simulink model "uz_pmsm_model_old_commit"  (R2023b)
settings: Solver=FixedStepAuto  StartTime=0.0  StopTime=0.05  RelTol=1e-3
PreLoadFcn:
  | uz_pmsm_model_init_parameter
PostLoadFcn:
  | % Import the data from Excel for a lookup table
  | FluxMapData = readtable('C:\Users\Philipp\ultrazohm\ultrazohm_sw\ip_cores\uz_pmsm_model\FluxMapData_2023-05-26_13-07-57.csv');
  | % Row indices for lookup table
  | d_current_in_d_axis = FluxMapData(8:27,1:end);
  | % Column indices for lookup table
  | q_current_in_d_axis = FluxMapData(29:48,1:end);
  | % Output values for lookup table
  | d_Flux_d_axis = FluxMapData(50:69,1:end);
values from neighbouring files (symbols this model uses):
  ad1 = ad_1(1)    [LUT_approx_methode2a.m]    (also in LUT_approx_methode2a_clean.m = ad_self(1); LUT_approx_methode_2a_FEM.m; fitting_parameter.mat = 0.03048394862; fitting_parameter_48V_SynRM.mat = 0.0218446789236)
  ad2 = ad_1(2)    [LUT_approx_methode2a.m]    (also in LUT_approx_methode2a_clean.m = ad_self(2); LUT_approx_methode_2a_FEM.m; fitting_parameter.mat = 0.0402440194669; fitting_parameter_48V_SynRM.mat = 0.015691946268)
  ad3 = ad_1(3)    [LUT_approx_methode2a.m]    (also in LUT_approx_methode2a_clean.m = ad_self(3); LUT_approx_methode_2a_FEM.m; fitting_parameter.mat = -16.4812001193; fitting_parameter_48V_SynRM.mat = 2.77465564774)
  ad4 = ad_3_6(1)    [LUT_approx_methode2a.m]    (also in LUT_approx_methode2a_clean.m = ad_4_6(1); LUT_approx_methode_2a_FEM.m; fitting_parameter.mat = 1.2964378241; fitting_parameter_48V_SynRM.mat = 0.0214529395212)
  ad5 = ad_3_6(2)    [LUT_approx_methode2a.m]    (also in LUT_approx_methode2a_clean.m = ad_4_6(2); LUT_approx_methode_2a_FEM.m; fitting_parameter.mat = 0.000618316734858; fitting_parameter_48V_SynRM.mat = 0.0128514742508)
  ad6 = ad_3_6(3)    [LUT_approx_methode2a.m]    (also in LUT_approx_methode2a_clean.m = ad_4_6(3); LUT_approx_methode_2a_FEM.m; fitting_parameter.mat = -12.2755860444; fitting_parameter_48V_SynRM.mat = 2.54408267654)
  aq1 = aq_1(1)    [LUT_approx_methode2a.m]    (also in LUT_approx_methode2a_clean.m = aq_self(1); LUT_approx_methode_2a_FEM.m; fitting_parameter.mat = 0.0048166705291; fitting_parameter_48V_SynRM.mat = 0.00205546577039)
  aq2 = aq_1(2)    [LUT_approx_methode2a.m]    (also in LUT_approx_methode2a_clean.m = aq_self(2); LUT_approx_methode_2a_FEM.m; fitting_parameter.mat = 0.171595255564; fitting_parameter_48V_SynRM.mat = 0.0602932843871)
  aq3 = aq_1(3)    [LUT_approx_methode2a.m]    (also in LUT_approx_methode2a_clean.m = aq_self(3); LUT_approx_methode_2a_FEM.m; fitting_parameter.mat = 0.000926293864031; fitting_parameter_48V_SynRM.mat = 4.42738872822e-05)
  aq4 = aq_3_6(1)    [LUT_approx_methode2a.m]    (also in LUT_approx_methode2a_clean.m = aq_4_6(1); LUT_approx_methode_2a_FEM.m; fitting_parameter.mat = 0.00500187099075; fitting_parameter_48V_SynRM.mat = 0.000698420875152)
  aq5 = aq_3_6(2)    [LUT_approx_methode2a.m]    (also in LUT_approx_methode2a_clean.m = aq_4_6(2); LUT_approx_methode_2a_FEM.m; fitting_parameter.mat = 0.17052123489; fitting_parameter_48V_SynRM.mat = 0.0493122483219)
  aq6 = aq_3_6(3)    [LUT_approx_methode2a.m]    (also in LUT_approx_methode2a_clean.m = aq_4_6(3); LUT_approx_methode_2a_FEM.m; fitting_parameter.mat = 0.00091860845; fitting_parameter_48V_SynRM.mat = 4.14644316065e-05)
  d_current_d_Flux = FluxMapData{1,1:20}    [uz_pmsm_model_init_parameter.m]
  d_current_q_Flux = FluxMapData{66,1:20}    [uz_pmsm_model_init_parameter.m]
  entkopplung_dynamic = false    [compare_simulation_to_measurement.m]    (also in uz_pmsm_model_init_parameter.m; uz_pmsm_model_init_parameter_clean.m)
  entkopplung_linear = true    [compare_simulation_to_measurement.m]    (also in uz_pmsm_model_init_parameter.m = false; uz_pmsm_model_init_parameter_clean.m = false)
  entkopplung_static = false    [compare_simulation_to_measurement.m]    (also in uz_pmsm_model_init_parameter.m = true; uz_pmsm_model_init_parameter_clean.m)
  Fid1_Giq1 = ((1/2).*(aq3-aq6).*((q_current_set).^2))+((aq1./aq2).*log(cosh(aq2.*q_current_set)))-((aq4/aq5).*log(cosh(aq5.*q_current_set)))    [LUT_approx_methode2a.m]    (also in LUT_approx_methode2a_clean.m; LUT_approx_methode_2a_FEM.m = (1/2).*(aq3-aq6).*((q_current_set).^2)+((aq1./aq2).*log(cosh; fitting_parameter.mat = -0.00135679401385; fitting_parameter_48V_SynRM.mat = 0.221350145237)
  Fid2_Giq2 = ((ad1./ad2).*(log(cosh(ad2.*(d_current_set-ad3))))) - ((ad4./ad5).*(log(cosh(ad5.*(d_current_set-ad6)))))    [LUT_approx_methode2a.m]    (also in LUT_approx_methode2a_clean.m; LUT_approx_methode_2a_FEM.m = ((ad1./ad2).*(log(cosh(ad2.*(d_current_set-ad3))))) - (((ad1; fitting_parameter.mat = 0.0788137932988; fitting_parameter_48V_SynRM.mat = 0.221214979406)
  Flux_d = FluxMapData{43:62,1:20}'*(1e-3)    [uz_pmsm_model_init_parameter.m]
  Flux_q = FluxMapData{108:127,1:20}'*(1e-3)    [uz_pmsm_model_init_parameter.m]
  friction_coefficient = 0.001    [uz_pmsm_model_init_parameter.m]    (also in uz_pmsm_model_init_parameter_clean.m)
  inertia = 0.000084    (= 8.4e-05)    [uz_pmsm_model_init_parameter.m]    (also in uz_pmsm_model_init_parameter_clean.m)
  L_d = 0.3    [uz_pmsm_model_init_parameter.m]    (also in uz_pmsm_model_init_parameter_clean.m = 0.00045)
  L_q = 0.3    [uz_pmsm_model_init_parameter.m]    (also in uz_pmsm_model_init_parameter_clean.m = 0.002)
  load_torque = 0    [uz_pmsm_model_init_parameter.m]
  parameter_nachfuerung = false    [compare_simulation_to_measurement.m]    (also in uz_pmsm_model_init_parameter.m; uz_pmsm_model_init_parameter_clean.m)
  polepair = 4    [uz_pmsm_model_init_parameter.m]    (also in uz_pmsm_model_init_parameter_clean.m)
  praediktion_entkopplung_nonlinear = false    [compare_simulation_to_measurement.m]    (also in uz_pmsm_model_init_parameter.m; uz_pmsm_model_init_parameter_clean.m = true)
  psi_pm = 0.0075    [uz_pmsm_model_init_parameter.m]    (also in uz_pmsm_model_init_parameter_clean.m = 0.0194)
  q_current_d_Flux = FluxMapData{22:41,1}    [uz_pmsm_model_init_parameter.m]
  q_current_q_Flux = FluxMapData{87:106,1}    [uz_pmsm_model_init_parameter.m]
  R_1 = 0.08    [uz_pmsm_model_init_parameter.m]    (also in uz_pmsm_model_init_parameter_clean.m = 0.3)
  rpm = 1250    [uz_pmsm_model_init_parameter.m]
  setpoint_step = 4.0    (= 4)    [compare_simulation_to_measurement.m]    (also in export_csv.m = 10; iae_von_cil_measurements.m = 8; uz_pmsm_model_init_parameter.m = 8; uz_pmsm_model_init_parameter_clean.m = 10)
  simulate_mechanical = true    [compare_simulation_to_measurement.m]    (also in export_csv.m = false; uz_pmsm_model_init_parameter.m = false; uz_pmsm_model_init_parameter_clean.m = false)
  simulate_nonlinear_modell = false    [compare_simulation_to_measurement.m]    (also in uz_pmsm_model_init_parameter.m = true; uz_pmsm_model_init_parameter_clean.m = true)
  simulate_open_loop = true    [compare_simulation_to_measurement.m]    (also in export_csv.m; uz_pmsm_model_init_parameter.m = false; uz_pmsm_model_init_parameter_clean.m = false)
  static_friction_torque = 0.01    [uz_pmsm_model_init_parameter.m]    (also in uz_pmsm_model_init_parameter_clean.m)
  tau_sum = 2*ts_regler    (= 0.0001)    [uz_pmsm_model_init_parameter.m]    (also in uz_pmsm_model_init_parameter_clean.m = 8e-05)
  ts = logs{k}.Values    [export_csv.m]    (also in uz_pmsm_model_init_parameter.m = 2e-06; uz_pmsm_model_init_parameter_clean.m = 2e-06)
  ts_regler = 1/20e3    (= 5e-05)    [uz_pmsm_model_init_parameter.m]    (also in uz_pmsm_model_init_parameter_clean.m = 4e-05)
undefined symbols (not defined in the file or in its folder): Ki_Bo_d, Ki_Bo_q, Kp_Bo_d, Kp_Bo_q, Ldq
libraries: slpidlib x6
(part 4 of 5)

== system uz_pmsm_model_old_commit/Curren t_Controller_With_FluxMaps_OLD/Psi_d_q2/psid_approx ==
  Id : Inport
  Iq : Inport  Port=2
  FittingParameters : Inport  Port=3
  Demux : Demux  Outputs=23
  Log : Math  Operator=log  SignedPower=on
  Log1 : Math  Operator=log  SignedPower=on
  Product{,1..2,4..5,8} (6 alike) : Product  OutDataTypeStr=Inherit: Same as first input
  Product10 : Product  Inputs=3
  Product{3,6..7,12} (4 alike) : Product
  Sum : Sum  Inputs=|+-  OutDataTypeStr=Inherit: Same as first input
  Sum1 : Sum  Inputs=|+-
  Sum2 : Sum  Inputs=|+-  OutDataTypeStr=Inherit: Same as first input
  Sum3 : Sum  Inputs=|++-  OutDataTypeStr=Inherit: Same as first input
  Sum7 : Sum  Inputs=|+-  OutDataTypeStr=Inherit: Same as first input
  Tanh : Trigonometry  Operator=tanh
  Tanh1 : Trigonometry  Operator=tanh
  Tanh2 : Trigonometry  Operator=cosh
  Tanh3 : Trigonometry  Operator=cosh
  Terminator : Terminator
  psid : Outport
  psiq_cross_s1_integrated : Outport  Port=2
  wires:
  FittingParameters/1 -> Demux/1
  Demux/1 -> Product1/2  "ad1"
  Demux/3 -> Sum/2  "ad3"
  Sum/1 -> Product/1
  Demux/2 -> Product/2  "ad2"
  Product1/1 -> Sum7/1, Sum2/1  "psidself"
  Demux/4 -> Product3/2  "ad4"
  Sum1/1 -> Product2/1
  Demux/5 -> Product2/2  "ad5"
  Demux/6 -> Sum1/2  "ad6"
  Id/1 -> Sum1/1, Sum/1
  Product3/1 -> Sum2/2  "psid_s1"
  Iq/1 -> Product8/2, Product8/1, Product5/1, Product4/1
  Sum2/1 -> Product10/1  "psid_cross_s1"
  Tanh2/1 -> Log/1
  Tanh3/1 -> Log1/1
  Product8/1 -> Product7/1
  Product7/1 -> Sum3/2
  Demux/20 -> Product6/2
  Product6/1 -> Sum3/1
  Demux/19 -> Product12/2
  Product12/1 -> Sum3/3
  Sum3/1 -> Product10/2, psiq_cross_s1_integrated/1  "psiq_cross_s1_integrated"
  Demux/11 -> Product5/2  "aq5"
  Demux/8 -> Product4/2  "aq2"
  Product10/1 -> Sum7/2  "psid_cross"
  Sum7/1 -> psid/1  "psi_d_approx"
  Demux/14 -> Terminator/1
  Demux/13 -> Product10/3  "Reciprodical_F1G1"
  Log/1 -> Product6/1
  Log1/1 -> Product12/1
  Tanh/1 -> Product1/1
  Tanh1/1 -> Product3/1
  Product/1 -> Tanh/1
  Product2/1 -> Tanh1/1
  Product4/1 -> Tanh2/1
  Product5/1 -> Tanh3/1
  Demux/23 -> Product7/2

== system uz_pmsm_model_old_commit/Curren t_Controller_With_FluxMaps_OLD/Psi_d_q2/psid_approx1 ==
  Id : Inport
  Iq : Inport  Port=2
  FittingParameters : Inport  Port=3
  Demux : Demux  Outputs=23
  Log : Math  Operator=log  SignedPower=on
  Log1 : Math  Operator=log  SignedPower=on
  Product{,1..2,4..5,8} (6 alike) : Product  OutDataTypeStr=Inherit: Same as first input
  Product10 : Product  Inputs=3
  Product{3,6..7,12} (4 alike) : Product
  Sum : Sum  Inputs=|+-  OutDataTypeStr=Inherit: Same as first input
  Sum1 : Sum  Inputs=|+-
  Sum2 : Sum  Inputs=|+-  OutDataTypeStr=Inherit: Same as first input
  Sum3 : Sum  Inputs=|++-  OutDataTypeStr=Inherit: Same as first input
  Sum7 : Sum  Inputs=|+-  OutDataTypeStr=Inherit: Same as first input
  Tanh : Trigonometry  Operator=tanh
  Tanh1 : Trigonometry  Operator=tanh
  Tanh2 : Trigonometry  Operator=cosh
  Tanh3 : Trigonometry  Operator=cosh
  Terminator : Terminator
  psid : Outport
  psiq_cross_s1_integrated : Outport  Port=2
  wires:
  FittingParameters/1 -> Demux/1
  Demux/1 -> Product1/2  "ad1"
  Demux/3 -> Sum/2  "ad3"
  Sum/1 -> Product/1
  Demux/2 -> Product/2  "ad2"
  Product1/1 -> Sum7/1, Sum2/1  "psidself"
  Demux/4 -> Product3/2  "ad4"
  Sum1/1 -> Product2/1
  Demux/5 -> Product2/2  "ad5"
  Demux/6 -> Sum1/2  "ad6"
  Id/1 -> Sum1/1, Sum/1
  Product3/1 -> Sum2/2  "psid_s1"
  Iq/1 -> Product8/2, Product8/1, Product5/1, Product4/1
  Sum2/1 -> Product10/1  "psid_cross_s1"
  Tanh2/1 -> Log/1
  Tanh3/1 -> Log1/1
  Product8/1 -> Product7/1
  Product7/1 -> Sum3/2
  Demux/20 -> Product6/2
  Product6/1 -> Sum3/1
  Demux/19 -> Product12/2
  Product12/1 -> Sum3/3
  Sum3/1 -> Product10/2, psiq_cross_s1_integrated/1  "psiq_cross_s1_integrated"
  Demux/11 -> Product5/2  "aq5"
  Demux/8 -> Product4/2  "aq2"
  Product10/1 -> Sum7/2  "psid_cross"
  Sum7/1 -> psid/1  "psi_d_approx"
  Demux/14 -> Terminator/1
  Demux/13 -> Product10/3  "Reciprodical_F1G1"
  Log/1 -> Product6/1
  Log1/1 -> Product12/1
  Tanh/1 -> Product1/1
  Tanh1/1 -> Product3/1
  Product/1 -> Tanh/1
  Product2/1 -> Tanh1/1
  Product4/1 -> Tanh2/1
  Product5/1 -> Tanh3/1
  Demux/23 -> Product7/2

== system uz_pmsm_model_old_commit/Curren t_Controller_With_FluxMaps_OLD/Psi_d_q2/psiq_approx ==
  Id : Inport
  Iq : Inport  Port=2
  FittingParameters : Inport  Port=3
  Demux : Demux  Outputs=23
  Log1 : Math  Operator=log  SignedPower=on
  Log2 : Math  Operator=log  SignedPower=on
  Product{,2,7,10} (4 alike) : Product  OutDataTypeStr=Inherit: Same as first input
  Product{1,3..6,9} (6 alike) : Product
  Product20 : Product  Inputs=3
  Sum1 : Sum  Inputs=|++
  Sum10 : Sum  Inputs=|+-
  Sum2 : Sum  Inputs=|+-
  Sum3 : Sum  Inputs=-+|
  Sum4 : Sum  Inputs=++|
  Sum5 : Sum  Inputs=|+-
  Sum6 : Sum  Inputs=-+|
  Tanh : Trigonometry  Operator=tanh
  Tanh1 : Trigonometry  Operator=tanh
  Tanh2 : Trigonometry  Operator=cosh
  Tanh4 : Trigonometry  Operator=cosh
  psiq : Outport
  psid_cross_s1_integrated : Outport  Port=2
  wires:
  FittingParameters/1 -> Demux/1
  Sum2/1 -> Product20/1  "psiq_cross_s1"
  Demux/10 -> Product3/2  "aq4"
  Demux/12 -> Product6/2  "aq6"
  Demux/8 -> Product/2  "aq2"
  Demux/11 -> Product2/2  "aq5"
  Demux/7 -> Product1/2  "aq1"
  Iq/1 -> Product2/1, Product6/1, Product/1, Product5/1
  Demux/9 -> Product5/2  "aq3"
  Tanh4/1 -> Log2/1
  Demux/22 -> Product4/1
  Product1/1 -> Sum4/2
  Product5/1 -> Sum4/1
  Sum4/1 -> Sum10/1, Sum2/1  "psiq_self"
  Sum1/1 -> Sum2/2
  Product3/1 -> Sum1/1  "psiq_s1"
  Product6/1 -> Sum1/2
  Sum3/1 -> Product7/2  "psid_cross_s1"
  Product7/1 -> Tanh4/1  "psid_s1"
  Product4/1 -> Sum5/1
  Product9/1 -> Sum5/2
  Product10/1 -> Tanh2/1  "psid_s1"
  Tanh2/1 -> Log1/1
  Demux/21 -> Product9/1
  Sum6/1 -> Product10/2  "psid_cross_s1"
  Demux/3 -> Sum3/1  "ad3"
  Demux/2 -> Product7/1  "ad2"
  Demux/5 -> Product10/1  "ad5"
  Demux/6 -> Sum6/1  "ad6"
  Id/1 -> Sum6/2, Sum3/2
  Sum5/1 -> psid_cross_s1_integrated/1, Product20/2  "psid_cross_s1_integrated"
  Product20/1 -> Sum10/2  "psiq_cross"
  Sum10/1 -> psiq/1  "psiq_approx"
  Demux/14 -> Product20/3
  Log1/1 -> Product9/2
  Log2/1 -> Product4/2
  Tanh1/1 -> Product3/1
  Tanh/1 -> Product1/1
  Product2/1 -> Tanh1/1
  Product/1 -> Tanh/1

== system uz_pmsm_model_old_commit/Curren t_Controller_With_FluxMaps_OLD/Psi_d_q2/psiq_approx1 ==
  Id : Inport
  Iq : Inport  Port=2
  FittingParameters : Inport  Port=3
  Demux : Demux  Outputs=23
  Log1 : Math  Operator=log  SignedPower=on
  Log2 : Math  Operator=log  SignedPower=on
  Product{,2,7,10} (4 alike) : Product  OutDataTypeStr=Inherit: Same as first input
  Product{1,3..6,9} (6 alike) : Product
  Product20 : Product  Inputs=3
  Sum1 : Sum  Inputs=|++
  Sum10 : Sum  Inputs=|+-  OutDataTypeStr=Inherit: Same as first input
  Sum2 : Sum  Inputs=|+-
  Sum3 : Sum  Inputs=-+|
  Sum4 : Sum  Inputs=++|
  Sum5 : Sum  Inputs=|+-
  Sum6 : Sum  Inputs=-+|
  Tanh : Trigonometry  Operator=tanh
  Tanh1 : Trigonometry  Operator=tanh
  Tanh2 : Trigonometry  Operator=cosh
  Tanh4 : Trigonometry  Operator=cosh
  psiq : Outport
  psid_cross_s1_integrated : Outport  Port=2
  wires:
  FittingParameters/1 -> Demux/1
  Sum2/1 -> Product20/1  "psiq_cross_s1"
  Demux/10 -> Product3/2  "aq4"
  Demux/12 -> Product6/2  "aq6"
  Demux/8 -> Product/2  "aq2"
  Demux/11 -> Product2/2  "aq5"
  Demux/7 -> Product1/2  "aq1"
  Iq/1 -> Product2/1, Product6/1, Product/1, Product5/1
  Demux/9 -> Product5/2  "aq3"
  Tanh4/1 -> Log2/1
  Demux/22 -> Product4/1
  Product1/1 -> Sum4/2
  Product5/1 -> Sum4/1
  Sum4/1 -> Sum10/1, Sum2/1  "psiq_self"
  Sum1/1 -> Sum2/2
  Product3/1 -> Sum1/1  "psiq_s1"
  Product6/1 -> Sum1/2
  Sum3/1 -> Product7/2  "psid_cross_s1"
  Product7/1 -> Tanh4/1  "psid_s1"
  Product4/1 -> Sum5/1
  Product9/1 -> Sum5/2
  Product10/1 -> Tanh2/1  "psid_s1"
  Tanh2/1 -> Log1/1
  Demux/21 -> Product9/1
  Sum6/1 -> Product10/2  "psid_cross_s1"
  Demux/3 -> Sum3/1  "ad3"
  Demux/2 -> Product7/1  "ad2"
  Demux/5 -> Product10/1  "ad5"
  Demux/6 -> Sum6/1  "ad6"
  Id/1 -> Sum6/2, Sum3/2
  Sum5/1 -> psid_cross_s1_integrated/1, Product20/2  "psid_cross_s1_integrated"
  Product20/1 -> Sum10/2  "psiq_cross"
  Sum10/1 -> psiq/1  "psiq_approx"
  Demux/14 -> Product20/3
  Log1/1 -> Product9/2
  Log2/1 -> Product4/2
  Tanh1/1 -> Product3/1
  Tanh/1 -> Product1/1
  Product2/1 -> Tanh1/1
  Product/1 -> Tanh/1

== system uz_pmsm_model_old_commit/Current_Controller1/Entkopplungen/Lineare_Entkopplung ==
  i_d : Inport
  i_q : Inport  Port=2
  omega_m : Inport  Port=3
  Constant1 : Constant  Value=psi_pm  OutDataTypeStr=Inherit: Inherit via back propagation  SampleTime=-1
  Gain : Gain  Gain=L_q
  Gain1 : Gain  Gain=L_d
  Gain2 : Gain  Gain=polepair  OutDataTypeStr=Inherit: Same as input
  Product : Product  OutDataTypeStr=Inherit: Same as first input
  Product1 : Product  OutDataTypeStr=Inherit: Same as first input
  Sum6 : Sum  Inputs=|++
  u_d : Outport
  u_q : Outport  Port=2
  wires:
  omega_m/1 -> Gain2/1
  Sum6/1 -> Product1/1
  Product/1 -> u_d/1
  i_d/1 -> Gain1/1
  i_q/1 -> Gain/1
  Product1/1 -> u_q/1
  Gain1/1 -> Sum6/1
  Gain2/1 -> Product1/2, Product/2
  Gain/1 -> Product/1
  Constant1/1 -> Sum6/2  "u_q"

== system uz_pmsm_model_old_commit/Current_Controller1/Entkopplungen/decoupling_praediktion ==
  i_d : Inport
  u_d_1 : Inport  Port=2
  i_q : Inport  Port=3
  u_q_1 : Inport  Port=4
  omega_m : Inport  Port=5
  u_d_k : Inport  Port=6
  u_q_k : Inport  Port=7
  psi_q : Inport  Port=8
  psi_d : Inport  Port=9
  Gain : Gain  Gain=R_1
  Gain1 : Gain  Gain=R_1
  Gain2 : Gain  Gain=polepair
  Gain3 : Gain  Gain=ts_regler
  Gain4 : Gain  Gain=ts_regler
  Gain5 : Gain  Gain=ts_regler/2
  Gain6 : Gain  Gain=ts_regler/2
  Product{1..4} (4 alike) : Product
  Sum : Sum  Inputs=|+-
  Sum1 : Sum  Inputs=|+-
  Sum2 : Sum  Inputs=++|
  Sum3 : Sum  Inputs=|-+
  Sum4 : Sum  Inputs=++|
  Sum5 : Sum  Inputs=|++
  Sum6 : Sum  Inputs=++|
  Sum7 : Sum  Inputs=|++
  u_d_entk : Outport
  u_q_entk : Outport  Port=2
  wires:
  psi_q/1 -> Sum5/2, Product2/1
  psi_d/1 -> Product3/2, Sum4/1
  Gain2/1 -> Product1/2, Product4/1, Product3/1, Product2/2
  u_d_k/1 -> Sum/2
  Gain/1 -> Sum/1
  u_q_k/1 -> Sum1/1
  Gain1/1 -> Sum1/2
  Product3/1 -> Sum3/1
  Product2/1 -> Sum2/2
  Sum/1 -> Sum2/1
  Sum1/1 -> Sum3/2
  Sum3/1 -> Gain4/1
  Sum2/1 -> Gain3/1
  Gain3/1 -> Sum4/2
  Gain4/1 -> Sum5/1
  u_d_1/1 -> Gain5/1
  Sum4/1 -> Sum6/2
  u_q_1/1 -> Gain6/1
  Gain5/1 -> Sum6/1
  Sum5/1 -> Sum7/1
  Gain6/1 -> Sum7/2
  Sum6/1 -> Product1/1
  Sum7/1 -> Product4/2
  omega_m/1 -> Gain2/1
  i_d/1 -> Gain/1
  i_q/1 -> Gain1/1
  Product1/1 -> u_q_entk/1
  Product4/1 -> u_d_entk/1

== system uz_pmsm_model_old_commit/Current_Controller1/Entkopplungen/dynamic_nonlinear_entkopplung1 ==
  i_d : Inport
  i_q : Inport  Port=2
  psi_d : Inport  Port=3
  psi_q : Inport  Port=4
  Ldq_LUT : Inport  Port=5
  Lqd_LUT : Inport  Port=6
  omega_m : Inport  Port=7
  Gain2 : Gain  Gain=polepair
  Product : Product  OutDataTypeStr=Inherit: Same as first input
  Product1 : Product  OutDataTypeStr=Inherit: Same as first input
  Product2 : Product
  Product3 : Product
  Sum1 : Sum  Inputs=++|  OutDataTypeStr=Inherit: Same as first input
  Sum6 : Sum  Inputs=++|
  u_d : Outport
  u_q : Outport  Port=2
  wires:
  psi_q/1 -> Product/1  "psi_q_LUT"
  Gain2/1 -> Product1/2, Product/2
  psi_d/1 -> Product1/1  "psi_d_LUT"
  omega_m/1 -> Gain2/1
  i_d/1 -> Product2/1
  Ldq_LUT/1 -> Product2/2
  Sum6/1 -> u_q/1
  Product1/1 -> Sum6/2
  Product/1 -> Sum1/2
  Sum1/1 -> u_d/1
  i_q/1 -> Product3/1
  Lqd_LUT/1 -> Product3/2
  Product3/1 -> Sum6/1
  Product2/1 -> Sum1/1

== system uz_pmsm_model_old_commit/Current_Controller1/Entkopplungen/static_nonlinear_entkopplung ==
  psi_d : Inport
  psi_q : Inport  Port=2
  omega_m : Inport  Port=3
  Gain2 : Gain  Gain=polepair
  Product : Product  OutDataTypeStr=Inherit: Same as first input
  Product1 : Product  OutDataTypeStr=Inherit: Same as first input
  u_d : Outport
  u_q : Outport  Port=2
  wires:
  psi_q/1 -> Product/1  "psi_q_LUT"
  Gain2/1 -> Product1/2, Product/2
  Product1/1 -> u_q/1
  Product/1 -> u_d/1
  psi_d/1 -> Product1/1  "psi_d_LUT"
  omega_m/1 -> Gain2/1

== system uz_pmsm_model_old_commit/Current_Controller1/Psi_d_q1/Ldd_approx1 ==
  psiq_cross_s1_integrated : Inport
  Id : Inport  Port=2
  FittingParameters : Inport  Port=3
  Demux : Demux  Outputs=23
  Product{,1..3} (4 alike) : Product  OutDataTypeStr=single
  Product10 : Product  Inputs=3  OutDataTypeStr=single
  Product14 : Product
  Product15 : Product
  Reciprocal : Product  Inputs=/  RndMeth=Zero  SaturateOnIntegerOverflow=on
  Reciprocal1 : Product  Inputs=/  RndMeth=Zero  SaturateOnIntegerOverflow=on
  Sum : Sum  Inputs=|+-  OutDataTypeStr=single
  Sum1 : Sum  Inputs=|+-  OutDataTypeStr=single
  Sum2 : Sum  Inputs=|+-
  Sum7 : Sum  Inputs=|+-
  Tanh1 : Trigonometry  Operator=cosh
  Tanh4 : Trigonometry  Operator=cosh
  Ldd : Outport
  wires:
  FittingParameters/1 -> Demux/1
  Demux/3 -> Sum/2  "ad3"
  Sum/1 -> Product/1
  Demux/2 -> Product/2  "ad2"
  Product1/1 -> Sum7/1, Sum2/1  "psidself_abgeleitet"
  Sum1/1 -> Product2/1
  Demux/5 -> Product2/2  "ad5"
  Demux/6 -> Sum1/2  "ad6"
  Id/1 -> Sum1/1, Sum/1
  Product3/1 -> Sum2/2  "psid_s1"
  Sum2/1 -> Product10/1  "psid_cross_s1_abgeleitet"
  Product10/1 -> Sum7/2  "psid_cross"
  Sum7/1 -> Ldd/1  "psid_cross_s1"
  Demux/13 -> Product10/3  "F1G1"
  Tanh4/1 -> Product14/1, Product14/2
  Tanh1/1 -> Product15/2, Product15/1
  Reciprocal1/1 -> Product3/1
  Product15/1 -> Reciprocal1/1
  Product14/1 -> Reciprocal/1
  Product/1 -> Tanh4/1
  Product2/1 -> Tanh1/1
  psiq_cross_s1_integrated/1 -> Product10/2
  Reciprocal/1 -> Product1/1
  Demux/15 -> Product3/2  "ad4*ad5"
  Demux/16 -> Product1/2  "ad1*ad2"

== system uz_pmsm_model_old_commit/Current_Controller1/Psi_d_q1/Lqq_approx1 ==
  psid_cross_s1_integrated : Inport
  Iq : Inport  Port=2
  FittingParameters : Inport  Port=3
  Demux : Demux  Outputs=23
  Product : Product  OutDataTypeStr=Inherit: Same as first input
  Product1 : Product
  Product14 : Product  OutDataTypeStr=Inherit: Same as first input
  Product15 : Product
  Product2 : Product  OutDataTypeStr=Inherit: Same as first input
  Product20 : Product  Inputs=3
  Product3 : Product
  Reciprocal : Product  Inputs=/  RndMeth=Zero  SaturateOnIntegerOverflow=on
  Reciprocal1 : Product  Inputs=/  RndMeth=Zero  SaturateOnIntegerOverflow=on
  Sum1 : Sum  Inputs=|++
  Sum10 : Sum  Inputs=|+-
  Sum2 : Sum  Inputs=|+-
  Sum4 : Sum  Inputs=|++
  Tanh1 : Trigonometry  Operator=cosh
  Tanh3 : Trigonometry  Operator=cosh
  Lqq : Outport
  wires:
  FittingParameters/1 -> Demux/1
  Demux/12 -> Sum4/2  "aq6"
  Product20/1 -> Sum10/2  "psiq_cross"
  Sum10/1 -> Lqq/1  "Lqq"
  Demux/14 -> Product20/3
  Demux/9 -> Sum1/2  "aq3"
  Tanh3/1 -> Product14/1, Product14/2
  Tanh1/1 -> Product15/2, Product15/1
  Sum2/1 -> Product20/1
  Reciprocal/1 -> Product1/1
  Reciprocal1/1 -> Product3/1
  Demux/8 -> Product/2  "aq2"
  Iq/1 -> Product2/1, Product/1
  Demux/11 -> Product2/2  "aq5"
  Product1/1 -> Sum1/1  "psidself_abgeleitet"
  Sum1/1 -> Sum10/1, Sum2/1
  Sum4/1 -> Sum2/2
  Product3/1 -> Sum4/1  "psid_s1"
  Product15/1 -> Reciprocal1/1
  Product2/1 -> Tanh1/1
  Product/1 -> Tanh3/1
  Product14/1 -> Reciprocal/1
  psid_cross_s1_integrated/1 -> Product20/2
  Demux/18 -> Product1/2  "aq1*aq2"
  Demux/17 -> Product3/2  "aq4*aq5"

== system uz_pmsm_model_old_commit/Current_Controller1/Psi_d_q1/psid_approx ==
  Id : Inport
  Iq : Inport  Port=2
  FittingParameters : Inport  Port=3
  Demux : Demux  Outputs=23
  Log : Math  Operator=log  SignedPower=on
  Log1 : Math  Operator=log  SignedPower=on
  Product{,1..2,4..5,8} (6 alike) : Product  OutDataTypeStr=Inherit: Same as first input
  Product10 : Product  Inputs=3
  Product{3,6..7,12} (4 alike) : Product
  Sum : Sum  Inputs=|+-  OutDataTypeStr=Inherit: Same as first input
  Sum1 : Sum  Inputs=|+-
  Sum2 : Sum  Inputs=|+-  OutDataTypeStr=Inherit: Same as first input
  Sum3 : Sum  Inputs=|++-  OutDataTypeStr=Inherit: Same as first input
  Sum7 : Sum  Inputs=|+-  OutDataTypeStr=Inherit: Same as first input
  Tanh : Trigonometry  Operator=tanh
  Tanh1 : Trigonometry  Operator=tanh
  Tanh2 : Trigonometry  Operator=cosh
  Tanh3 : Trigonometry  Operator=cosh
  Terminator : Terminator
  psid : Outport
  psiq_cross_s1_integrated : Outport  Port=2
  wires:
  FittingParameters/1 -> Demux/1
  Demux/1 -> Product1/2  "ad1"
  Demux/3 -> Sum/2  "ad3"
  Sum/1 -> Product/1
  Demux/2 -> Product/2  "ad2"
  Product1/1 -> Sum7/1, Sum2/1  "psidself"
  Demux/4 -> Product3/2  "ad4"
  Sum1/1 -> Product2/1
  Demux/5 -> Product2/2  "ad5"
  Demux/6 -> Sum1/2  "ad6"
  Id/1 -> Sum1/1, Sum/1
  Product3/1 -> Sum2/2  "psid_s1"
  Iq/1 -> Product8/2, Product8/1, Product5/1, Product4/1
  Sum2/1 -> Product10/1  "psid_cross_s1"
  Tanh2/1 -> Log/1
  Tanh3/1 -> Log1/1
  Product8/1 -> Product7/1
  Product7/1 -> Sum3/2
  Demux/20 -> Product6/2
  Product6/1 -> Sum3/1
  Demux/19 -> Product12/2
  Product12/1 -> Sum3/3
  Sum3/1 -> Product10/2, psiq_cross_s1_integrated/1  "psiq_cross_s1_integrated"
  Demux/11 -> Product5/2  "aq5"
  Demux/8 -> Product4/2  "aq2"
  Product10/1 -> Sum7/2  "psid_cross"
  Sum7/1 -> psid/1  "psi_d_approx"
  Demux/14 -> Terminator/1
  Demux/13 -> Product10/3  "Reciprodical_F1G1"
  Log/1 -> Product6/1
  Log1/1 -> Product12/1
  Tanh/1 -> Product1/1
  Tanh1/1 -> Product3/1
  Product/1 -> Tanh/1
  Product2/1 -> Tanh1/1
  Product4/1 -> Tanh2/1
  Product5/1 -> Tanh3/1
  Demux/23 -> Product7/2

== system uz_pmsm_model_old_commit/Current_Controller1/Psi_d_q1/psiq_approx ==
  Id : Inport
  Iq : Inport  Port=2
  FittingParameters : Inport  Port=3
  Demux : Demux  Outputs=23
  Log1 : Math  Operator=log  SignedPower=on
  Log2 : Math  Operator=log  SignedPower=on
  Product{,2,7,10} (4 alike) : Product  OutDataTypeStr=Inherit: Same as first input
  Product{1,3..6,9} (6 alike) : Product
  Product20 : Product  Inputs=3
  Sum1 : Sum  Inputs=|++
  Sum10 : Sum  Inputs=|+-
  Sum2 : Sum  Inputs=|+-
  Sum3 : Sum  Inputs=-+|
  Sum4 : Sum  Inputs=++|
  Sum5 : Sum  Inputs=|+-
  Sum6 : Sum  Inputs=-+|
  Tanh : Trigonometry  Operator=tanh
  Tanh1 : Trigonometry  Operator=tanh
  Tanh2 : Trigonometry  Operator=cosh
  Tanh4 : Trigonometry  Operator=cosh
  psiq : Outport
  psid_cross_s1_integrated : Outport  Port=2
  wires:
  FittingParameters/1 -> Demux/1
  Sum2/1 -> Product20/1  "psiq_cross_s1"
  Demux/10 -> Product3/2  "aq4"
  Demux/12 -> Product6/2  "aq6"
  Demux/8 -> Product/2  "aq2"
  Demux/11 -> Product2/2  "aq5"
  Demux/7 -> Product1/2  "aq1"
  Iq/1 -> Product2/1, Product6/1, Product/1, Product5/1
  Demux/9 -> Product5/2  "aq3"
  Tanh4/1 -> Log2/1
  Demux/22 -> Product4/1
  Product1/1 -> Sum4/2
  Product5/1 -> Sum4/1
  Sum4/1 -> Sum10/1, Sum2/1  "psiq_self"
  Sum1/1 -> Sum2/2
  Product3/1 -> Sum1/1  "psiq_s1"
  Product6/1 -> Sum1/2
  Sum3/1 -> Product7/2  "psid_cross_s1"
  Product7/1 -> Tanh4/1  "psid_s1"
  Product4/1 -> Sum5/1
  Product9/1 -> Sum5/2
  Product10/1 -> Tanh2/1  "psid_s1"
  Tanh2/1 -> Log1/1
  Demux/21 -> Product9/1
  Sum6/1 -> Product10/2  "psid_cross_s1"
  Demux/3 -> Sum3/1  "ad3"
  Demux/2 -> Product7/1  "ad2"
  Demux/5 -> Product10/1  "ad5"
  Demux/6 -> Sum6/1  "ad6"
  Id/1 -> Sum6/2, Sum3/2
  Sum5/1 -> psid_cross_s1_integrated/1, Product20/2  "psid_cross_s1_integrated"
  Product20/1 -> Sum10/2  "psiq_cross"
  Sum10/1 -> psiq/1  "psiq_approx"
  Demux/14 -> Product20/3
  Log1/1 -> Product9/2
  Log2/1 -> Product4/2
  Tanh1/1 -> Product3/1
  Tanh/1 -> Product1/1
  Product2/1 -> Tanh1/1
  Product/1 -> Tanh/1

== system uz_pmsm_model_old_commit/Current_Controller_With_FluxMaps_OLD1/Entkopplungen/Lineare_Entkopplung ==
  i_d : Inport
  i_q : Inport  Port=2
  omega_m : Inport  Port=3
  Constant1 : Constant  Value=psi_pm  SampleTime=-1
  Gain : Gain  Gain=L_q
  Gain1 : Gain  Gain=L_d
  Gain2 : Gain  Gain=polepair  OutDataTypeStr=Inherit: Same as input
  Product : Product
  Product1 : Product
  Sum6 : Sum  Inputs=|++
  u_d : Outport
  u_q : Outport  Port=2
  wires:
  omega_m/1 -> Gain2/1
  Sum6/1 -> Product1/1
  Product/1 -> u_d/1
  i_d/1 -> Gain1/1
  Constant1/1 -> Sum6/2
  i_q/1 -> Gain/1
  Product1/1 -> u_q/1
  Gain1/1 -> Sum6/1
  Gain2/1 -> Product1/2, Product/2
  Gain/1 -> Product/1

== system uz_pmsm_model_old_commit/Current_Controller_With_FluxMaps_OLD1/Entkopplungen/decoupling_praediktion ==
  i_d : Inport
  u_d_1 : Inport  Port=2
  i_q : Inport  Port=3
  u_q_1 : Inport  Port=4
  omega_m : Inport  Port=5
  u_d_k : Inport  Port=6
  u_q_k : Inport  Port=7
  psi_q : Inport  Port=8
  psi_d : Inport  Port=9
  Gain : Gain  Gain=R_1
  Gain1 : Gain  Gain=R_1
  Gain2 : Gain  Gain=polepair
  Gain3 : Gain  Gain=ts_regler
  Gain4 : Gain  Gain=ts_regler
  Gain5 : Gain  Gain=ts_regler/2
  Gain6 : Gain  Gain=ts_regler/2
  Product{1..4} (4 alike) : Product
  Sum : Sum  Inputs=|+-
  Sum1 : Sum  Inputs=|+-
  Sum2 : Sum  Inputs=++|
  Sum3 : Sum  Inputs=|-+
  Sum4 : Sum  Inputs=++|
  Sum5 : Sum  Inputs=|++
  Sum6 : Sum  Inputs=++|
  Sum7 : Sum  Inputs=|++
  u_d_entk : Outport
  u_q_entk : Outport  Port=2
  wires:
  psi_q/1 -> Sum5/2, Product2/1
  psi_d/1 -> Product3/2, Sum4/1
  Gain2/1 -> Product1/2, Product4/1, Product3/1, Product2/2
  u_d_k/1 -> Sum/2
  Gain/1 -> Sum/1
  u_q_k/1 -> Sum1/1
  Gain1/1 -> Sum1/2
  Product3/1 -> Sum3/1
  Product2/1 -> Sum2/2
  Sum/1 -> Sum2/1
  Sum1/1 -> Sum3/2
  Sum3/1 -> Gain4/1
  Sum2/1 -> Gain3/1
  Gain3/1 -> Sum4/2
  Gain4/1 -> Sum5/1
  u_d_1/1 -> Gain5/1
  Sum4/1 -> Sum6/2
  u_q_1/1 -> Gain6/1
  Gain5/1 -> Sum6/1
  Sum5/1 -> Sum7/1
  Gain6/1 -> Sum7/2
  Sum6/1 -> Product1/1
  Sum7/1 -> Product4/2
  omega_m/1 -> Gain2/1
  i_d/1 -> Gain/1
  i_q/1 -> Gain1/1
  Product1/1 -> u_q_entk/1
  Product4/1 -> u_d_entk/1

== system uz_pmsm_model_old_commit/Current_Controller_With_FluxMaps_OLD1/Entkopplungen/dynamic_nonlinear_entkopplung1 ==
  i_d : Inport
  i_q : Inport  Port=2
  psi_d : Inport  Port=3
  psi_q : Inport  Port=4
  Ldq_LUT : Inport  Port=5
  Lqd_LUT : Inport  Port=6
  omega_m : Inport  Port=7
  Gain2 : Gain  Gain=polepair
  Product{,1..3} (4 alike) : Product
  Sum1 : Sum  Inputs=++|
  Sum6 : Sum  Inputs=++|
  u_d : Outport
  u_q : Outport  Port=2
  wires:
  psi_q/1 -> Product/1  "psi_q_LUT"
  Gain2/1 -> Product1/2, Product/2
  psi_d/1 -> Product1/1  "psi_d_LUT"
  omega_m/1 -> Gain2/1
  i_d/1 -> Product2/1
  Ldq_LUT/1 -> Product2/2
  Sum6/1 -> u_q/1
  Product1/1 -> Sum6/2
  Product/1 -> Sum1/2
  Sum1/1 -> u_d/1
  i_q/1 -> Product3/1
  Lqd_LUT/1 -> Product3/2
  Product3/1 -> Sum6/1
  Product2/1 -> Sum1/1

== system uz_pmsm_model_old_commit/Current_Controller_With_FluxMaps_OLD1/Entkopplungen/static_nonlinear_entkopplung ==
  psi_d : Inport
  psi_q : Inport  Port=2
  omega_m : Inport  Port=3
  Gain2 : Gain  Gain=polepair
  Product : Product
  Product1 : Product
  Scope : Scope  NumInputPorts=2
  u_d : Outport
  u_q : Outport  Port=2
  wires:
  psi_q/1 -> Product/1  "psi_q_LUT"
  Gain2/1 -> Product1/2, Product/2
  Product1/1 -> Scope/1, u_q/1
  Product/1 -> Scope/2, u_d/1
  psi_d/1 -> Product1/1  "psi_d_LUT"
  omega_m/1 -> Gain2/1

== system uz_pmsm_model_old_commit/uz_pmsm_model/mechanical_system/integrator1 ==
  reset : Inport
  in : Inport  Port=2
  Delay1 : Delay  DelayLength=1  ExternalReset=Level
      settings: InputPortMap=u0,r5
  Gain : Gain  Gain=ts
  Sum3 : Sum  Inputs=|++
  outt : Outport
  wires:
  in/1 -> Gain/1
  Gain/1 -> Sum3/1
  reset/1 -> Delay1/2
  Sum3/1 -> Delay1/1
  Delay1/1 -> Sum3/2, outt/1

== system uz_pmsm_model_old_commit/uz_pmsm_model/pmsm/Ldd_approx1 ==
  Id : Inport
  psiq_cross_s1_integrated : Inport  Port=2
  FittingParameters : Inport  Port=3
  Constant2 : Constant  Value="eps(\"single\")"  OutDataTypeStr=single  SampleTime=ts
  Demux : Demux  Outputs=23
  Product{,1..3} (4 alike) : Product  OutDataTypeStr=single
  Product10 : Product  Inputs=3  OutDataTypeStr=single
  Product14 : Product
  Product15 : Product
  Reciprocal : Product  Inputs=/  RndMeth=Zero  SaturateOnIntegerOverflow=on
  Reciprocal1 : Product  Inputs=/  RndMeth=Zero  SaturateOnIntegerOverflow=on
  Sum : Sum  Inputs=|+-  OutDataTypeStr=single
  Sum1 : Sum  Inputs=|+-  OutDataTypeStr=single
  Sum2 : Sum  Inputs=|+-
  Sum7 : Sum  Inputs=|+-
  Switch : Switch  Criteria=u2 ~= 0  Threshold="eps(\"single\")"  SaturateOnIntegerOverflow=off  InputSameDT=off
  Switch1 : Switch  Criteria=u2 ~= 0  Threshold="eps(\"single\")"  SaturateOnIntegerOverflow=off  InputSameDT=off
  Tanh1 : Trigonometry  Operator=cosh
  Tanh4 : Trigonometry  Operator=cosh
  Ldd : Outport
  wires:
  FittingParameters/1 -> Demux/1
  Demux/3 -> Sum/2  "ad3"
  Sum/1 -> Product/1
  Demux/2 -> Product/2  "ad2"
  Product1/1 -> Sum7/1, Sum2/1  "psidself_abgeleitet"
  Sum1/1 -> Product2/1
  Demux/5 -> Product2/2  "ad5"
  Demux/6 -> Sum1/2  "ad6"
  Id/1 -> Sum1/1, Sum/1
  Product3/1 -> Sum2/2  "psid_s1"
  Sum2/1 -> Product10/1  "psid_cross_s1_abgeleitet"
  Product10/1 -> Sum7/2  "psid_cross"
  Sum7/1 -> Ldd/1  "psid_cross_s1"
  Demux/13 -> Product10/3  "F1G1"
  Tanh4/1 -> Product14/1, Product14/2
  Tanh1/1 -> Product15/1, Product15/2
  Reciprocal1/1 -> Product3/1
  Product/1 -> Tanh4/1
  Product2/1 -> Tanh1/1
  psiq_cross_s1_integrated/1 -> Product10/2
  Reciprocal/1 -> Product1/1
  Demux/15 -> Product3/2  "ad4*ad5"
  Demux/16 -> Product1/2  "ad1*ad2"
  Product14/1 -> Switch/1, Switch/2
  Constant2/1 -> Switch/3, Switch1/3
  Switch/1 -> Reciprocal/1
  Product15/1 -> Switch1/1, Switch1/2
  Switch1/1 -> Reciprocal1/1

== system uz_pmsm_model_old_commit/uz_pmsm_model/pmsm/Ldq ==
  psid_cross_s1 : Inport
  psiq_cross_s1 : Inport  Port=2
  FittingParameters : Inport  Port=3
  Gain : Gain  Gain=-1
  Product20 : Product  Inputs=3
  Selector : Selector  InputPortWidth=23  IndexOptions=Index vector (dialog)  Indices=[13]  OutputSizes=1
  psiq : Outport
  wires:
  Product20/1 -> Gain/1  "psiq_cross"
  psid_cross_s1/1 -> Product20/1
  Gain/1 -> psiq/1
  psiq_cross_s1/1 -> Product20/2
  FittingParameters/1 -> Selector/1
  Selector/1 -> Product20/3

== system uz_pmsm_model_old_commit/uz_pmsm_model/pmsm/Lqd ==
  psid_cross_s1 : Inport
  psiq_cross_s1 : Inport  Port=2
  FittingParameters : Inport  Port=3
  Gain : Gain  Gain=-1
  Product20 : Product  Inputs=3
  Selector : Selector  InputPortWidth=23  IndexOptions=Index vector (dialog)  Indices=[14]  OutputSizes=1
  Lqd : Outport
  wires:
  FittingParameters/1 -> Selector/1
  Product20/1 -> Gain/1
  psid_cross_s1/1 -> Product20/1
  Gain/1 -> Lqd/1
  psiq_cross_s1/1 -> Product20/2
  Selector/1 -> Product20/3

== system uz_pmsm_model_old_commit/uz_pmsm_model/pmsm/Lqq_approx1 ==
  psid_cross_s1_integrated : Inport
  Iq : Inport  Port=2
  FittingParameters : Inport  Port=3
  Constant2 : Constant  Value="eps(\"single\")"  OutDataTypeStr=single  SampleTime=ts
  Demux : Demux  Outputs=23
  Product : Product  OutDataTypeStr=Inherit: Same as first input
  Product{1,3,14..15} (4 alike) : Product
  Product2 : Product  OutDataTypeStr=Inherit: Same as first input
  Product20 : Product  Inputs=3
  Reciprocal : Product  Inputs=/  RndMeth=Zero  SaturateOnIntegerOverflow=on
  Reciprocal1 : Product  Inputs=/  RndMeth=Zero  SaturateOnIntegerOverflow=on
  Sum1 : Sum  Inputs=|++
  Sum10 : Sum  Inputs=|+-
  Sum2 : Sum  Inputs=|+-
  Sum4 : Sum  Inputs=|++
  Switch : Switch  Criteria=u2 ~= 0  Threshold="eps(\"single\")"  SaturateOnIntegerOverflow=off  InputSameDT=off
  Switch1 : Switch  Criteria=u2 ~= 0  Threshold="eps(\"single\")"  SaturateOnIntegerOverflow=off  InputSameDT=off
  Tanh1 : Trigonometry  Operator=cosh
  Tanh3 : Trigonometry  Operator=cosh
  Lqq : Outport
  wires:
  FittingParameters/1 -> Demux/1
  Demux/12 -> Sum4/2  "aq6"
  Product20/1 -> Sum10/2  "psiq_cross"
  Sum10/1 -> Lqq/1  "Lqq"
  Demux/14 -> Product20/3
  Demux/9 -> Sum1/2  "aq3"
  Tanh3/1 -> Product14/1, Product14/2
  Tanh1/1 -> Product15/2, Product15/1
  Sum2/1 -> Product20/1
  Reciprocal/1 -> Product1/1
  Reciprocal1/1 -> Product3/1
  Demux/8 -> Product/2  "aq2"
  Iq/1 -> Product2/1, Product/1
  Demux/11 -> Product2/2  "aq5"
  Product1/1 -> Sum1/1  "psidself_abgeleitet"
  Sum1/1 -> Sum10/1, Sum2/1
  Sum4/1 -> Sum2/2
  Product3/1 -> Sum4/1  "psid_s1"
  Product2/1 -> Tanh1/1
  Product/1 -> Tanh3/1
  psid_cross_s1_integrated/1 -> Product20/2
  Demux/18 -> Product1/2  "aq1*aq2"
  Demux/17 -> Product3/2  "aq4*aq5"
  Product14/1 -> Switch/2, Switch/1
  Constant2/1 -> Switch/3, Switch1/3
  Switch/1 -> Reciprocal/1
  Product15/1 -> Switch1/2, Switch1/1
  Switch1/1 -> Reciprocal1/1

== system uz_pmsm_model_old_commit/uz_pmsm_model/pmsm/Subsystem ==
  in : Inport
  reset : Inport  Port=2
  Delay1 : Delay  DelayLength=1  ExternalReset=Level
      settings: InputPortMap=u0,r5
  Gain7 : Gain  Gain=ts
  Sum5 : Sum  Inputs=|++  OutDataTypeStr=Inherit: Same as first input
  outt : Outport
  wires:
  in/1 -> Gain7/1
  reset/1 -> Delay1/2
  Delay1/1 -> outt/1, Sum5/2
  Sum5/1 -> Delay1/1
  Gain7/1 -> Sum5/1  "u_d"

== system uz_pmsm_model_old_commit/uz_pmsm_model/pmsm/Subsystem1 ==
  in : Inport
  reset : Inport  Port=2
  Delay1 : Delay  DelayLength=1  ExternalReset=Level
      settings: InputPortMap=u0,r5
  Gain7 : Gain  Gain=ts
  Sum5 : Sum  Inputs=|++
  outt : Outport
  wires:
  in/1 -> Gain7/1
  reset/1 -> Delay1/2
  Delay1/1 -> outt/1, Sum5/2
  Sum5/1 -> Delay1/1
  Gain7/1 -> Sum5/1  "u_d"

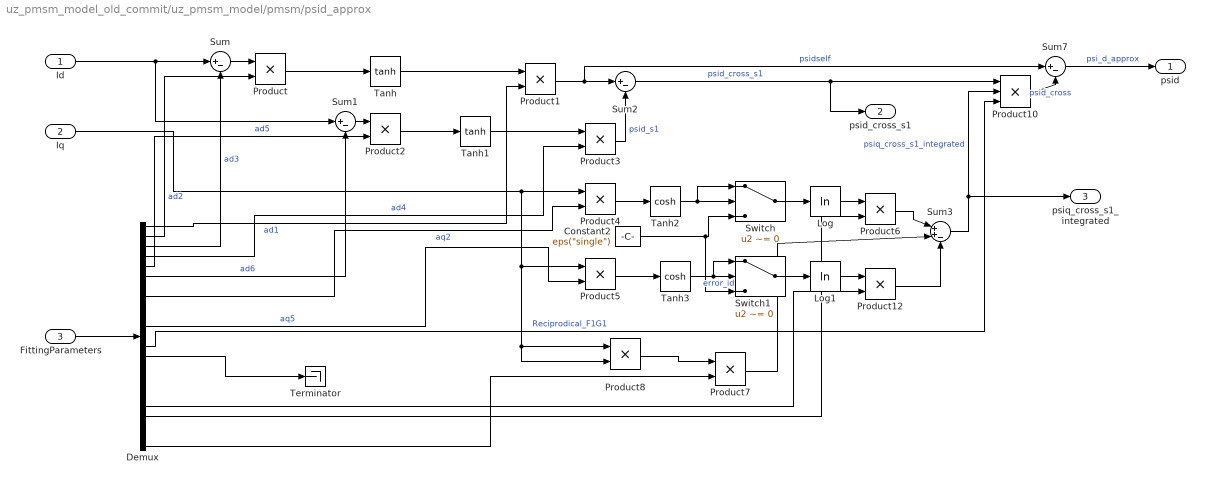
== system uz_pmsm_model_old_commit/uz_pmsm_model/pmsm/psid_approx ==
  Id : Inport
  Iq : Inport  Port=2
  FittingParameters : Inport  Port=3
  Constant2 : Constant  Value="eps(\"single\")"  OutDataTypeStr=single  SampleTime=ts
  Demux : Demux  Outputs=23
  Log : Math  Operator=log  SignedPower=on
  Log1 : Math  Operator=log  SignedPower=on
  Product{,2,4..5,8} (5 alike) : Product  OutDataTypeStr=Inherit: Same as first input
  Product{1,3,6..7,12} (5 alike) : Product
  Product10 : Product  Inputs=3
  Sum{,1..2,7} (4 alike) : Sum  Inputs=|+-
  Sum3 : Sum  Inputs=|++-
  Switch : Switch  Criteria=u2 ~= 0  Threshold="eps(\"single\")"  SaturateOnIntegerOverflow=off  InputSameDT=off
  Switch1 : Switch  Criteria=u2 ~= 0  Threshold="eps(\"single\")"  SaturateOnIntegerOverflow=off  InputSameDT=off
  Tanh : Trigonometry  Operator=tanh
  Tanh1 : Trigonometry  Operator=tanh
  Tanh2 : Trigonometry  Operator=cosh
  Tanh3 : Trigonometry  Operator=cosh
  Terminator : Terminator
  psid : Outport
  psid_cross_s1 : Outport  Port=2
  psiq_cross_s1_integrated : Outport  Port=3
  wires:
  FittingParameters/1 -> Demux/1
  Demux/1 -> Product1/2  "ad1"
  Demux/3 -> Sum/2  "ad3"
  Sum/1 -> Product/1
  Demux/2 -> Product/2  "ad2"
  Product1/1 -> Sum7/1, Sum2/1  "psidself"
  Demux/4 -> Product3/2  "ad4"
  Sum1/1 -> Product2/1
  Demux/5 -> Product2/2  "ad5"
  Demux/6 -> Sum1/2  "ad6"
  Id/1 -> Sum1/1, Sum/1
  Product3/1 -> Sum2/2  "psid_s1"
  Iq/1 -> Product8/2, Product8/1, Product5/1, Product4/1
  Sum2/1 -> psid_cross_s1/1, Product10/1  "psid_cross_s1"
  Product8/1 -> Product7/1
  Product7/1 -> Sum3/2
  Demux/20 -> Product6/2
  Product6/1 -> Sum3/1
  Demux/19 -> Product12/2
  Product12/1 -> Sum3/3
  Sum3/1 -> Product10/2, psiq_cross_s1_integrated/1  "psiq_cross_s1_integrated"
  Demux/11 -> Product5/2  "aq5"
  Demux/8 -> Product4/2  "aq2"
  Product10/1 -> Sum7/2  "psid_cross"
  Sum7/1 -> psid/1  "psi_d_approx"
  Demux/14 -> Terminator/1
  Demux/13 -> Product10/3  "Reciprodical_F1G1"
  Log/1 -> Product6/1
  Log1/1 -> Product12/1
  Tanh/1 -> Product1/1
  Tanh1/1 -> Product3/1
  Product/1 -> Tanh/1
  Product2/1 -> Tanh1/1
  Product4/1 -> Tanh2/1
  Product5/1 -> Tanh3/1
  Demux/23 -> Product7/2
  Tanh2/1 -> Switch/1, Switch/2
  Switch/1 -> Log/1
  Tanh3/1 -> Switch1/2, Switch1/1  "error_id"
  Constant2/1 -> Switch1/3, Switch/3
  Switch1/1 -> Log1/1

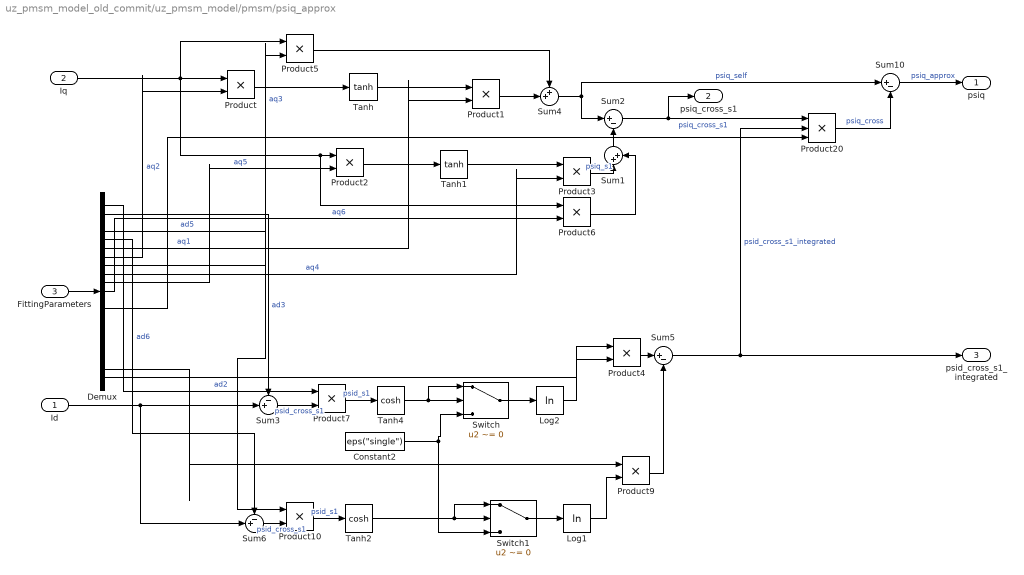
== system uz_pmsm_model_old_commit/uz_pmsm_model/pmsm/psiq_approx ==
  Id : Inport
  Iq : Inport  Port=2
  FittingParameters : Inport  Port=3
  Constant2 : Constant  Value="eps(\"single\")"  OutDataTypeStr=single  SampleTime=ts
  Demux : Demux  Outputs=23
  Log1 : Math  Operator=log  SignedPower=on
  Log2 : Math  Operator=log  SignedPower=on
  Product{,2,7,10} (4 alike) : Product  OutDataTypeStr=Inherit: Same as first input
  Product{1,3..6,9} (6 alike) : Product
  Product20 : Product  Inputs=3
  Sum1 : Sum  Inputs=|++
  Sum10 : Sum  Inputs=|+-
  Sum2 : Sum  Inputs=|+-
  Sum3 : Sum  Inputs=-+|
  Sum4 : Sum  Inputs=++|
  Sum5 : Sum  Inputs=|+-
  Sum6 : Sum  Inputs=-+|
  Switch : Switch  Criteria=u2 ~= 0  Threshold="eps(\"single\")"  SaturateOnIntegerOverflow=off  InputSameDT=off
  Switch1 : Switch  Criteria=u2 ~= 0  Threshold="eps(\"single\")"  SaturateOnIntegerOverflow=off  InputSameDT=off
  Tanh : Trigonometry  Operator=tanh
  Tanh1 : Trigonometry  Operator=tanh
  Tanh2 : Trigonometry  Operator=cosh
  Tanh4 : Trigonometry  Operator=cosh
  psiq : Outport
  psiq_cross_s1 : Outport  Port=2
  psid_cross_s1_integrated : Outport  Port=3
  wires:
  FittingParameters/1 -> Demux/1
  Sum2/1 -> Product20/1, psiq_cross_s1/1  "psiq_cross_s1"
  Demux/10 -> Product3/2  "aq4"
  Demux/12 -> Product6/2  "aq6"
  Demux/8 -> Product/2  "aq2"
  Demux/11 -> Product2/2  "aq5"
  Demux/7 -> Product1/2  "aq1"
  Iq/1 -> Product2/1, Product6/1, Product/1, Product5/1
  Demux/9 -> Product5/2  "aq3"
  Demux/22 -> Product4/1
  Product1/1 -> Sum4/2
  Product5/1 -> Sum4/1
  Sum4/1 -> Sum10/1, Sum2/1  "psiq_self"
  Sum1/1 -> Sum2/2
  Product3/1 -> Sum1/1  "psiq_s1"
  Product6/1 -> Sum1/2
  Sum3/1 -> Product7/2  "psid_cross_s1"
  Product7/1 -> Tanh4/1  "psid_s1"
  Product4/1 -> Sum5/1
  Product9/1 -> Sum5/2
  Product10/1 -> Tanh2/1  "psid_s1"
  Demux/21 -> Product9/1
  Sum6/1 -> Product10/2  "psid_cross_s1"
  Demux/3 -> Sum3/1  "ad3"
  Demux/2 -> Product7/1  "ad2"
  Demux/5 -> Product10/1  "ad5"
  Demux/6 -> Sum6/1  "ad6"
  Id/1 -> Sum6/2, Sum3/2
  Sum5/1 -> psid_cross_s1_integrated/1, Product20/2  "psid_cross_s1_integrated"
  Product20/1 -> Sum10/2  "psiq_cross"
  Sum10/1 -> psiq/1  "psiq_approx"
  Demux/14 -> Product20/3
  Log1/1 -> Product9/2
  Log2/1 -> Product4/2
  Tanh1/1 -> Product3/1
  Tanh/1 -> Product1/1
  Product2/1 -> Tanh1/1
  Product/1 -> Tanh/1
  Tanh4/1 -> Switch/1, Switch/2
  Switch/1 -> Log2/1
  Constant2/1 -> Switch/3, Switch1/3
  Tanh2/1 -> Switch1/1, Switch1/2
  Switch1/1 -> Log1/1

== system uz_pmsm_model_old_commit/Curren t_Controller_With_FluxMaps_OLD/#embedded-Coder/Psi_d_q/psid_approx ==
  Id : Inport
  Iq : Inport  Port=2
  FittingParameters : Inport  Port=3
  Demux : Demux  Outputs=23
  Log : Math  Operator=log  SignedPower=on
  Log1 : Math  Operator=log  SignedPower=on
  Product{,1..2,4..5,8} (6 alike) : Product  OutDataTypeStr=Inherit: Same as first input
  Product10 : Product  Inputs=3
  Product{3,6..7,12} (4 alike) : Product
  Sum : Sum  Inputs=|+-  OutDataTypeStr=Inherit: Same as first input
  Sum1 : Sum  Inputs=|+-
  Sum2 : Sum  Inputs=|+-  OutDataTypeStr=Inherit: Same as first input
  Sum3 : Sum  Inputs=|++-  OutDataTypeStr=Inherit: Same as first input
  Sum7 : Sum  Inputs=|+-  OutDataTypeStr=Inherit: Same as first input
  Tanh : Trigonometry  Operator=tanh
  Tanh1 : Trigonometry  Operator=tanh
  Tanh2 : Trigonometry  Operator=cosh
  Tanh3 : Trigonometry  Operator=cosh
  Terminator : Terminator
  psid : Outport
  wires:
  FittingParameters/1 -> Demux/1
  Demux/1 -> Product1/2  "ad1"
  Demux/3 -> Sum/2  "ad3"
  Sum/1 -> Product/1
  Demux/2 -> Product/2  "ad2"
  Product1/1 -> Sum7/1, Sum2/1  "psidself"
  Demux/4 -> Product3/2  "ad4"
  Sum1/1 -> Product2/1
  Demux/5 -> Product2/2  "ad5"
  Demux/6 -> Sum1/2  "ad6"
  Id/1 -> Sum1/1, Sum/1
  Product3/1 -> Sum2/2  "psid_s1"
  Iq/1 -> Product8/2, Product8/1, Product5/1, Product4/1
  Sum2/1 -> Product10/1  "psid_cross_s1"
  Tanh2/1 -> Log/1
  Tanh3/1 -> Log1/1
  Product8/1 -> Product7/1
  Product7/1 -> Sum3/2
  Demux/20 -> Product6/2
  Product6/1 -> Sum3/1
  Demux/19 -> Product12/2
  Product12/1 -> Sum3/3
  Sum3/1 -> Product10/2  "psiq_cross_s1_integrated"
  Demux/11 -> Product5/2  "aq5"
  Demux/8 -> Product4/2  "aq2"
  Product10/1 -> Sum7/2  "psid_cross"
  Sum7/1 -> psid/1  "psi_d_approx"
  Demux/14 -> Terminator/1
  Demux/13 -> Product10/3  "Reciprodical_F1G1"
  Log/1 -> Product6/1
  Log1/1 -> Product12/1
  Tanh/1 -> Product1/1
  Tanh1/1 -> Product3/1
  Product/1 -> Tanh/1
  Product2/1 -> Tanh1/1
  Product4/1 -> Tanh2/1
  Product5/1 -> Tanh3/1
  Demux/23 -> Product7/2

== system uz_pmsm_model_old_commit/Curren t_Controller_With_FluxMaps_OLD/#embedded-Coder/Psi_d_q/psid_approx1 ==
  Id : Inport
  Iq : Inport  Port=2
  FittingParameters : Inport  Port=3
  Demux : Demux  Outputs=23
  Log : Math  Operator=log  SignedPower=on
  Log1 : Math  Operator=log  SignedPower=on
  Product{,1..2,4..5,8} (6 alike) : Product  OutDataTypeStr=Inherit: Same as first input
  Product10 : Product  Inputs=3
  Product{3,6..7,12} (4 alike) : Product
  Sum : Sum  Inputs=|+-  OutDataTypeStr=Inherit: Same as first input
  Sum1 : Sum  Inputs=|+-
  Sum2 : Sum  Inputs=|+-  OutDataTypeStr=Inherit: Same as first input
  Sum3 : Sum  Inputs=|++-  OutDataTypeStr=Inherit: Same as first input
  Sum7 : Sum  Inputs=|+-  OutDataTypeStr=Inherit: Same as first input
  Tanh : Trigonometry  Operator=tanh
  Tanh1 : Trigonometry  Operator=tanh
  Tanh2 : Trigonometry  Operator=cosh
  Tanh3 : Trigonometry  Operator=cosh
  Terminator : Terminator
  psid : Outport
  wires:
  FittingParameters/1 -> Demux/1
  Demux/1 -> Product1/2  "ad1"
  Demux/3 -> Sum/2  "ad3"
  Sum/1 -> Product/1
  Demux/2 -> Product/2  "ad2"
  Product1/1 -> Sum7/1, Sum2/1  "psidself"
  Demux/4 -> Product3/2  "ad4"
  Sum1/1 -> Product2/1
  Demux/5 -> Product2/2  "ad5"
  Demux/6 -> Sum1/2  "ad6"
  Id/1 -> Sum1/1, Sum/1
  Product3/1 -> Sum2/2  "psid_s1"
  Iq/1 -> Product8/2, Product8/1, Product5/1, Product4/1
  Sum2/1 -> Product10/1  "psid_cross_s1"
  Tanh2/1 -> Log/1
  Tanh3/1 -> Log1/1
  Product8/1 -> Product7/1
  Product7/1 -> Sum3/2
  Demux/20 -> Product6/2
  Product6/1 -> Sum3/1
  Demux/19 -> Product12/2
  Product12/1 -> Sum3/3
  Sum3/1 -> Product10/2  "psiq_cross_s1_integrated"
  Demux/11 -> Product5/2  "aq5"
  Demux/8 -> Product4/2  "aq2"
  Product10/1 -> Sum7/2  "psid_cross"
  Sum7/1 -> psid/1  "psi_d_approx"
  Demux/14 -> Terminator/1
  Demux/13 -> Product10/3  "Reciprodical_F1G1"
  Log/1 -> Product6/1
  Log1/1 -> Product12/1
  Tanh/1 -> Product1/1
  Tanh1/1 -> Product3/1
  Product/1 -> Tanh/1
  Product2/1 -> Tanh1/1
  Product4/1 -> Tanh2/1
  Product5/1 -> Tanh3/1
  Demux/23 -> Product7/2

== system uz_pmsm_model_old_commit/Curren t_Controller_With_FluxMaps_OLD/#embedded-Coder/Psi_d_q/psiq_approx ==
  Id : Inport
  Iq : Inport  Port=2
  FittingParameters : Inport  Port=3
  Demux : Demux  Outputs=23
  Log1 : Math  Operator=log  SignedPower=on
  Log2 : Math  Operator=log  SignedPower=on
  Product{,2,7,10} (4 alike) : Product  OutDataTypeStr=Inherit: Same as first input
  Product{1,3..6,9} (6 alike) : Product
  Product20 : Product  Inputs=3
  Sum1 : Sum  Inputs=|++
  Sum10 : Sum  Inputs=|+-
  Sum2 : Sum  Inputs=|+-
  Sum3 : Sum  Inputs=-+|
  Sum4 : Sum  Inputs=++|
  Sum5 : Sum  Inputs=|+-
  Sum6 : Sum  Inputs=-+|
  Tanh : Trigonometry  Operator=tanh
  Tanh1 : Trigonometry  Operator=tanh
  Tanh2 : Trigonometry  Operator=cosh
  Tanh4 : Trigonometry  Operator=cosh
  psiq : Outport
  wires:
  FittingParameters/1 -> Demux/1
  Sum2/1 -> Product20/1  "psiq_cross_s1"
  Demux/10 -> Product3/2  "aq4"
  Demux/12 -> Product6/2  "aq6"
  Demux/8 -> Product/2  "aq2"
  Demux/11 -> Product2/2  "aq5"
  Demux/7 -> Product1/2  "aq1"
  Iq/1 -> Product2/1, Product6/1, Product/1, Product5/1
  Demux/9 -> Product5/2  "aq3"
  Tanh4/1 -> Log2/1
  Demux/22 -> Product4/1
  Product1/1 -> Sum4/2
  Product5/1 -> Sum4/1
  Sum4/1 -> Sum10/1, Sum2/1  "psiq_self"
  Sum1/1 -> Sum2/2
  Product3/1 -> Sum1/1  "psiq_s1"
  Product6/1 -> Sum1/2
  Sum3/1 -> Product7/2  "psid_cross_s1"
  Product7/1 -> Tanh4/1  "psid_s1"
  Product4/1 -> Sum5/1
  Product9/1 -> Sum5/2
  Product10/1 -> Tanh2/1  "psid_s1"
  Tanh2/1 -> Log1/1
  Demux/21 -> Product9/1
  Sum6/1 -> Product10/2  "psid_cross_s1"
  Demux/3 -> Sum3/1  "ad3"
  Demux/2 -> Product7/1  "ad2"
  Demux/5 -> Product10/1  "ad5"
  Demux/6 -> Sum6/1  "ad6"
  Id/1 -> Sum6/2, Sum3/2
  Sum5/1 -> Product20/2  "psid_cross_s1_integrated"
  Product20/1 -> Sum10/2  "psiq_cross"
  Sum10/1 -> psiq/1  "psiq_approx"
  Demux/14 -> Product20/3
  Log1/1 -> Product9/2
  Log2/1 -> Product4/2
  Tanh1/1 -> Product3/1
  Tanh/1 -> Product1/1
  Product2/1 -> Tanh1/1
  Product/1 -> Tanh/1
